simulink model "PlasmaGlucoseInsulin"  (R2023a)
settings: Solver=ode23  StartTime=0.0  StopTime=10  MaxStep=0.1  RelTol=1e-3  EnableMultiTasking=on
libraries: simulink x2
settings Model: Creator=SUDEEP
settings SolverCC: AlgebraicLoopSolver=TrustRegion
settings DataIOCC: LimitDataPoints=on  SaveFormat=Array  ReturnWorkspaceOutputs=off
settings OptimizationCC: LifeSpan=inf
settings DebuggingCC: UnderspecifiedInitializationDetection=Classic  MergeDetectMultiDrivingBlocksExec=none  SolverPrmCheckMsg=warning  UnconnectedInputMsg=warning  UnconnectedOutputMsg=warning  UnconnectedLineMsg=warning  StateNameClashWarn=warning  SFUnexpectedBacktrackingDiag=warning  SFNoUnconditionalDefaultTransitionDiag=warning  SFExecutionAtInitializationDiag=none  ArithmeticOperatorsInVariantConditions=warning
settings HardwareCC: ProdBitPerPointer=32  ProdBitPerSizeT=32  ProdBitPerPtrDiffT=32  ProdLargestAtomicFloat=None  ProdIntDivRoundTo=Undefined  ProdEndianess=Unspecified  ProdWordSize=32  ProdHWDeviceType=32-bit Generic
settings ModelReferenceCC: EnableRefExpFcnMdlSchedulingChecks=on  PropagateSignalLabelsOutOfModel=off
settings SFSimCC: SimUseLocalCustomCode=off  CustomCodeUndefinedFunction=UseInterfaceOnly
settings RTWCC: RTWUseLocalCustomCode=off
settings CodeAppCC: StateflowObjectComments=on
settings GRTTargetCC: TargetLangStandard=C89/C90 (ANSI)
settings ConfigComp: CovMetricSettings=dw  CovSaveCumulativeToWorkspaceVar=on  CovSaveSingleToWorkspaceVar=on  CovExternalEMLEnable=off

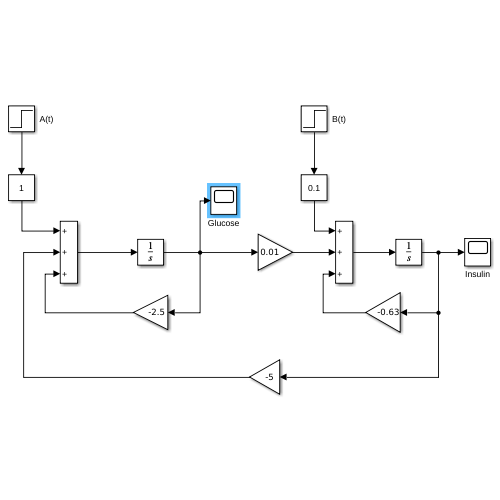
[thumbnail: Simulink's stored preview of the top-level diagram]
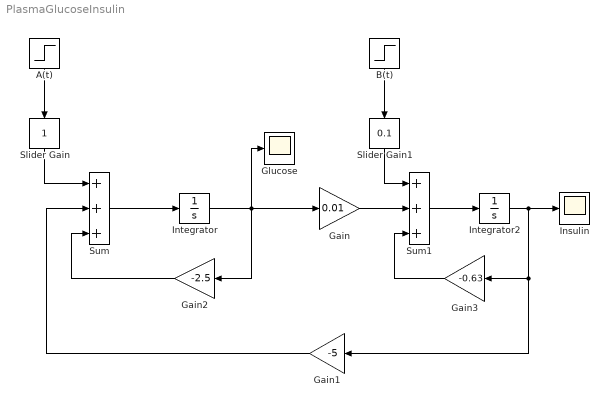
== system PlasmaGlucoseInsulin ==
  A(t) : Step  SampleTime=0
  B(t) : Step  Time=0  SampleTime=0
  Gain : Gain  Gain=0.01
  Gain1 : Gain  Gain=-5
  Gain2 : Gain  Gain=-2.5
  Gain3 : Gain  Gain=-0.63
  Glucose : Scope
  Insulin : Scope
  Integrator : Integrator
  Integrator2 : Integrator
  Slider Gain : simulink/Math Operations/Slider Gain  gain=1  low=0  high=2
  Slider Gain1 : simulink/Math Operations/Slider Gain  gain=0.1  low=0  high=2
  Sum : Sum  Inputs=+++
  Sum1 : Sum  Inputs=+++
  wires:
  A(t)/1 -> Slider Gain/1
  B(t)/1 -> Slider Gain1/1
  Sum/1 -> Integrator/1
  Integrator/1 -> Glucose/1, Gain2/1, Gain/1
  Gain/1 -> Sum1/2
  Sum1/1 -> Integrator2/1
  Slider Gain1/1 -> Sum1/1
  Gain1/1 -> Sum/2
  Gain3/1 -> Sum1/3
  Integrator2/1 -> Insulin/1, Gain1/1, Gain3/1
  Gain2/1 -> Sum/3
  Slider Gain/1 -> Sum/1
